simulink model "neural_net"  (R2015b)
settings: Solver=ode14x  StartTime=0.0  StopTime=inf  FixedStep=0.001  RelTol=1e-3
values from neighbouring files (symbols this model uses):
  A_aug = [A Bz; zeros(2,6)]    [Furuta_Pendulum_bring_down.m]    (also in Furuta_Pendulum_up_pos.m)
  B_aug = [B ;0;0]    [Furuta_Pendulum_bring_down.m]    (also in Furuta_Pendulum_up_pos.m)
  C_aug = [C zeros(2,2)]    [Furuta_Pendulum_bring_down.m]    (also in Furuta_Pendulum_up_pos.m)
  I_max = 0.5    [Furuta_Pendulum_bring_down.m]    (also in Furuta_Pendulum_up_pos.m = 0.8)
  Km = 7.86e-3    (= 0.00786)    [Furuta_Pendulum_bring_down.m]    (also in Furuta_Pendulum_up_pos.m)
  L_aug = real (L1+L2+L3)    [Furuta_Pendulum_bring_down.m]    (also in Furuta_Pendulum_up_pos.m)
  N = 70    [Furuta_Pendulum_bring_down.m]    (also in Furuta_Pendulum_up_pos.m)
  nu = 0.9    [Furuta_Pendulum_bring_down.m]    (also in Furuta_Pendulum_up_pos.m)
  R = 2.75    [Furuta_Pendulum_bring_down.m]    (also in Furuta_Pendulum_up_pos.m)
  V_max = 5    [Furuta_Pendulum_bring_down.m]    (also in Furuta_Pendulum_up_pos.m = 8)
undefined symbols (not defined in the file or in its folder): HIL, qc_get_step_size
libraries: quarc_library x5, simulink x1
settings Model: SimulationMode=external  ExtModeTrigDuration=10000  Creator=sgillen  LastModifiedBy=sgillen
settings SolverCC: PositivePriorityOrder=on
settings RTWCC: SystemTargetFile=quarc_win64.tlc  TemplateMakefile=quarc_default_tmf  Description=QUARC Win64 Target
settings STFCustomTargetCC: GeneratePreprocessorConditionals=Use local settings  CPPClassGenCompliant=off
settings GRTTargetCC: ParMdlRefBuildCompliant=off  CompOptLevelCompliant=off  CombineOutputUpdateFcns=off  MatFileLogging=off  CPPClassGenCompliant=off  GRTInterface=on  UseToolchainInfoCompliant=off  ExtMode=on  ExtModeMexFile=quarc_comm

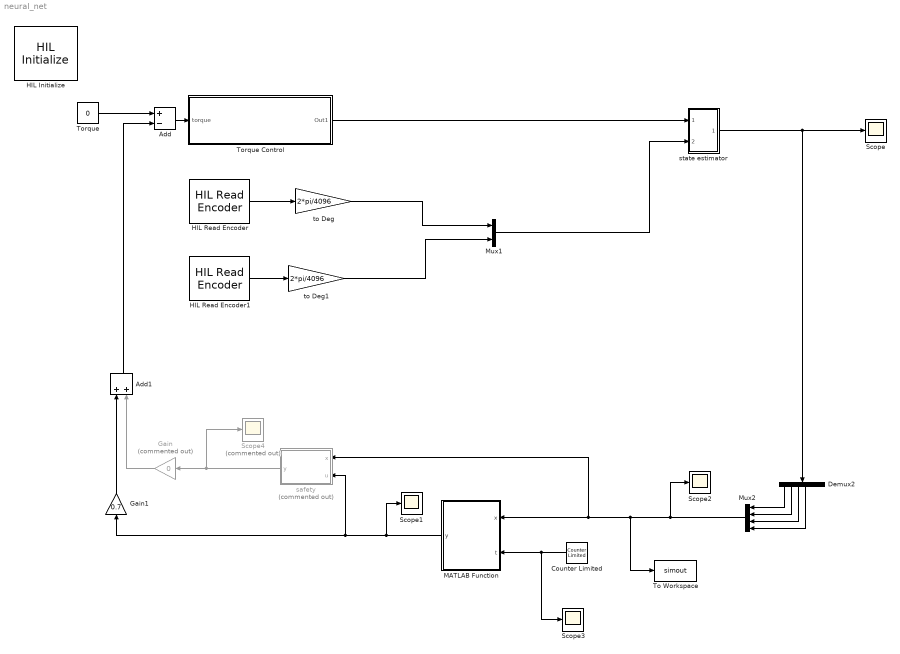
== system neural_net ==
  Add : Sum  Inputs=+-
  Add1 : Sum
  Counter Limited : simulink/Sources/Counter Limited  uplimit=.2/qc_get_step_size;  tsamp=-1
  Demux2 : Demux  Outputs=6
  Gain : Gain  Commented=on  Gain=0
  Gain1 : Gain  Gain=0.7
  HIL Initialize : quarc_library/Data Acquisition/Generic/Configuration/HIL Initialize  object_name=HIL-1  board_type=q4  board_number=0  board_options=""  exclusive=off  active=on  hardware_clocks=[0:1]  clock_modes=[0 0]  initial_clock_frequencies=[]  set_clock_params_at_start=on  set_clock_params_at_switch_in=off  set_clock_frequencies_at_start=off  set_clock_frequencies_at_switch_in=off  analog_input_channels=[0:3]  analog_input_configurations=[]  analog_input_maximums=10  analog_input_minimums=-10  set_analog_input_params_at_start=off  set_analog_input_params_at_switch_in=off  analog_output_channels=[0:3]  analog_output_maximums=[10]  analog_output_minimums=[-10]  initial_analog_outputs=[0]  final_analog_outputs=[0]  watchdog_analog_outputs=0  set_analog_output_params_at_start=on  set_analog_output_params_at_switch_in=off  set_analog_outputs_at_start=on  set_analog_outputs_at_switch_in=off  set_analog_outputs_at_terminate=on  set_analog_outputs_at_switch_out=off  set_analog_outputs_on_watchdog=off  digital_input_channels=[]  digital_output_channels=[]  digital_output_configuration=[]  initial_digital_outputs=[1]  final_digital_outputs=[1]  watchdog_digital_outputs=[2]  set_digital_output_params_at_start=off  set_digital_output_params_at_switch_in=off  set_digital_outputs_at_start=on  set_digital_outputs_at_switch_in=off  set_digital_outputs_at_terminate=on  set_digital_outputs_at_switch_out=off  set_digital_outputs_on_watchdog=off  encoder_channels=[0:3]  quadrature=[4]  encoder_filter_frequency=(1/60e-9)/1  initial_encoder_counts=[0]  set_encoder_params_at_start=on  set_encoder_params_at_switch_in=off  set_encoder_counts_at_start=on  set_encoder_counts_at_switch_in=off  pwm_channels=[]  pwm_modes=[0]  pwm_frequency=(1/60e-9)/1024  pwm_configuration=[]  pwm_alignment=[]  pwm_polarity=[]  pwm_leading_deadband=[]  pwm_trailing_deadband=[]  initial_pwm_outputs=[0]  final_pwm_outputs=[0]  watchdog_pwm_outputs=[]  set_pwm_params_at_start=on  set_pwm_params_at_switch_in=off  set_pwm_outputs_at_start=on  set_pwm_outputs_at_switch_in=off  set_pwm_outputs_at_terminate=on  set_pwm_outputs_at_switch_out=off  set_pwm_outputs_on_watchdog=off  other_output_channels=[]  initial_other_outputs=[]  final_other_outputs=[]  watchdog_other_outputs=[]  set_other_outputs_at_start=off  set_other_outputs_at_switch_in=off  set_other_outputs_at_terminate=off  set_other_outputs_at_switch_out=off  set_other_outputs_on_watchdog=off
  HIL Read Encoder : quarc_library/Data Acquisition/Generic/Immediate I//O/HIL Read Encoder  object_name=HIL-1  channels=0  sample_time=qc_get_step_size  active=on  vector_output=off  data_type_mode=Inherit via back propagation  data_type=double
  HIL Read Encoder1 : quarc_library/Data Acquisition/Generic/Immediate I//O/HIL Read Encoder  object_name=HIL-1  channels=1  sample_time=qc_get_step_size  active=on  vector_output=off  data_type_mode=Inherit via back propagation  data_type=double
  MATLAB Function : MATLAB Function  TreatAsAtomicUnit=on
  Mux1 : Mux  Inputs=2
  Mux2 : Mux
  Scope{,1..3} (4 alike) : Scope
  Scope4 : Scope  Commented=on
  To Workspace : ToWorkspace  VariableName=simout  SaveFormat=Timeseries  SampleTime=-1
  Torque : Constant  Value=0
  Torque Control : Subsystem
  safety : MATLAB Function  Commented=on  TreatAsAtomicUnit=on
  state estimator : Subsystem
  to Deg : Gain  Gain=2*pi/4096
  to Deg1 : Gain  Gain=2*pi/4096
  wires:
  HIL Read Encoder/1 -> to Deg/1
  HIL Read Encoder1/1 -> to Deg1/1
  to Deg1/1 -> Mux1/2
  to Deg/1 -> Mux1/1
  Demux2/1 -> Mux2/1
  Demux2/3 -> Mux2/3
  Demux2/2 -> Mux2/2
  Demux2/4 -> Mux2/4
  Torque/1 -> Add/1
  Add/1 -> Torque Control/1(torque)
  MATLAB Function/1(y) -> safety/2(u), Gain1/1, Scope1/1
  Torque Control/1(Out1) -> state estimator/1(In1)
  Mux1/1 -> state estimator/2(In2)
  state estimator/1(Out1) -> Demux2/1, Scope/1
  Mux2/1 -> Scope2/1, To Workspace/1, safety/1(x), MATLAB Function/1(x)
  Counter Limited/1 -> Scope3/1, MATLAB Function/2(t)
  safety/1(y) -> Gain/1, Scope4/1
  Gain1/1 -> Add1/1
  Add1/1 -> Add/2
  Gain/1 -> Add1/2

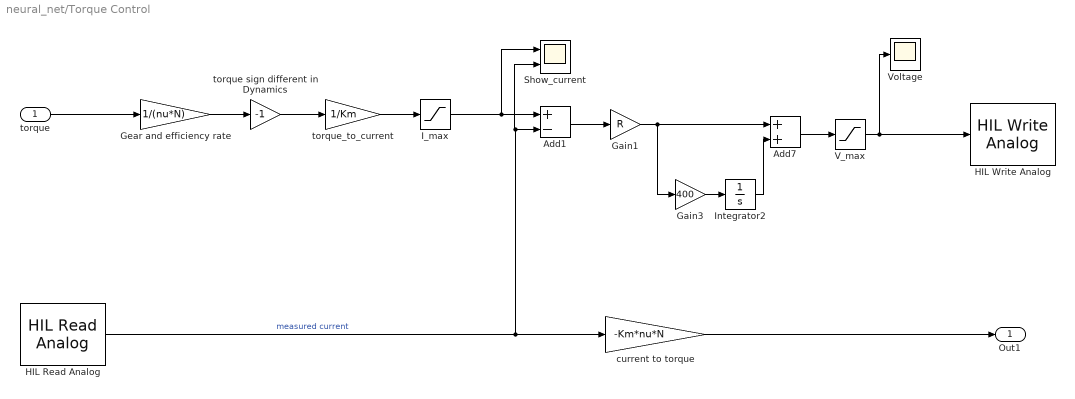
== system neural_net/Torque Control ==
  torque : Inport
  Add1 : Sum  Inputs=+-
  Add7 : Sum
  Gain1 : Gain  Gain=R
  Gain3 : Gain  Gain=400
  Gear and efficiency rate : Gain  Gain=1/(nu*N)
  HIL Read Analog : quarc_library/Data Acquisition/Generic/Immediate I//O/HIL Read Analog  object_name=HIL-1  channels=1  sample_time=qc_get_step_size  active=on  vector_output=off
  HIL Write Analog : quarc_library/Data Acquisition/Generic/Immediate I//O/HIL Write Analog  object_name=HIL-1  channels=0  sample_time=-1  active=off  vector_input=off
  I_max : Saturate  UpperLimit=I_max  LowerLimit=-I_max
  Integrator2 : Integrator
  Show_current : Scope  NumInputPorts=2
  V_max : Saturate  UpperLimit=V_max  LowerLimit=-V_max
  Voltage : Scope
  current to torque : Gain  Gain=-Km*nu*N
  torque sign different in Dynamics : Gain  Gain=-1
  torque_to_current : Gain  Gain=1/Km
  Out1 : Outport
  wires:
  Gear and efficiency rate/1 -> torque sign different in Dynamics/1
  HIL Read Analog/1 -> Add1/2, Show_current/2, current to torque/1  "measured current"
  Add1/1 -> Gain1/1
  torque sign different in Dynamics/1 -> torque_to_current/1
  Add7/1 -> V_max/1
  I_max/1 -> Show_current/1, Add1/1
  Gain3/1 -> Integrator2/1
  Gain1/1 -> Add7/1, Gain3/1
  V_max/1 -> Voltage/1, HIL Write Analog/1
  Integrator2/1 -> Add7/2
  torque_to_current/1 -> I_max/1
  current to torque/1 -> Out1/1
  torque/1 -> Gear and efficiency rate/1

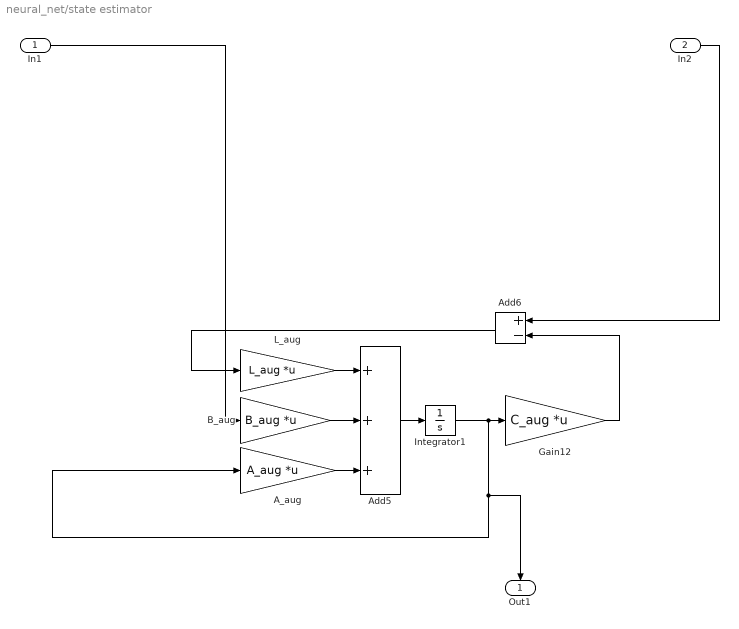
== system neural_net/state estimator ==
  In1 : Inport
  In2 : Inport  Port=2
  A_aug : Gain  Gain=A_aug  Multiplication=Matrix(K*u) (u vector)
  Add5 : Sum  Inputs=+++
  Add6 : Sum  Inputs=+-
  B_aug : Gain  Gain=B_aug  Multiplication=Matrix(K*u) (u vector)
  Gain12 : Gain  Gain=C_aug  Multiplication=Matrix(K*u) (u vector)
  Integrator1 : Integrator
  "L_aug " : Gain  Gain=L_aug  Multiplication=Matrix(K*u) (u vector)
  Out1 : Outport
  wires:
  Integrator1/1 -> Gain12/1, Out1/1, A_aug/1
  Add5/1 -> Integrator1/1
  In2/1 -> Add6/1
  Gain12/1 -> Add6/2
  Add6/1 -> "L_aug "/1
  A_aug/1 -> Add5/3
  B_aug/1 -> Add5/2
  "L_aug "/1 -> Add5/1
  In1/1 -> B_aug/1

== matlab function neural_net/safety ==
  data: x input; u input; y output
function y = fcn(x,u)
%% Parameter / Saturration
velocity_max = 1;
pos_max = 0.5 ; %pi/5
saturation = 0 ; % torque max is 0.2476 Nm

%%
phi1 = x(1);
phi2 = x(2);
vel1 = x(3); % velocity motor
vel2 = x(4); % velocity pendulum

 
if abs(phi1)>= pos_max % abs(vel1) >= velocity_max && 
    y = saturation;
    y = 0.2*sign(phi1)
else
    y = u;
end

== matlab function neural_net/MATLAB Function ==
  data: x input; y output; t input
function y = ffnn(x, t) % might make these global in a second...
%fully connected network
persistent w, persistent b
persistent obs_mat, persistent act_mat
persistent y_last, persistent t_persistent


fd = fopen('test.dat');
qc_get_step_size = 1e-3;
dt = 2;
frame_skip = dt/qc_get_step_size;

std = .1;
hsize = 24;
ep_length = 100;

num_weights = 2*(hsize^2) + hsize*5 + hsize*3 + 1

%% saturation, safety 
velocity_max = 1;
pos_max = 0.5 ; %pi/5
saturation = 0 ; % torque max is 0.2476 Nm
phi1 = x(1); % pos motor
vel1 = x(3); % velocity motor

%%
% init persistent state
% -------------------------------------
if isempty(w) || isempty(b) 
    w = {rand(4,hsize)/sqrt(num_weights), rand(hsize,hsize)/sqrt(num_weights), rand(hsize, hsize)/sqrt(num_weights), rand(hsize,1)/sqrt(num_weights)};
    b = {rand(hsize,1)/sqrt(num_weights), rand(hsize,1)/sqrt(num_weights), rand(hsize,1)/sqrt(num_weights), rand(1,1)/sqrt(num_weights)};
end
if isempty(obs_mat) || isempty(act_mat) 
    obs_mat = zeros(ep_length,4);
    act_mat = zeros(ep_length,1);
end

if isempty(t_persistent) || isempty(y_last)
    y_last =0;
    t_persistent =0;
end     

obs_mat(t+1,:) = x

if t == 1 && t_persistent~=t

    % do nn calculation
    % -------------------------------------

    size_w = size(w);
    num_layers = size_w(2);

    % xi = x';
    % for i = 1:num_layers-1
    %     xi = w{i}'*xi + b{i};
    %     xi = tanh(xi);
    % end


    %fine
    x1 = tanh(w{1}'*x + b{1})
    x2 = tanh(w{2}'*x1 + b{2})
    x3 = tanh(w{3}'*x2 + b{3})
    mean = w{end}'*x3;
    %mean = w{end}'*x3 + b{end};
    y = (randn*std + mean)
    y_last = y;
    
    if abs(phi1)>= pos_max % abs(vel1) >= velocity_max && 
        y = saturation;
        y = 0.2*sign(phi1)
        y_last = y
    end    

else
    y = y_last;
end

t_persistent = double(t);

% record obs and action (and logprob and state?)
% -------------------------------------
obs_mat(t+1,:) = x
act_mat(t+1,:) = y

end
